simulink model "DG1"  (R2020a)
settings: Solver=VariableStepAuto  StartTime=0.0  StopTime=20  RelTol=1e-3
values from neighbouring files (symbols this model uses):
  cf1 = 50 * 1e-6    (= 5e-05)    [parameters.m]
  F1 = 0.75    [parameters.m]
  kic1 = 16e3    (= 16000)    [parameters.m]
  kiv1 = 390    [parameters.m]
  kpc1 = 10.5    [parameters.m]
  kpv1 = 0.05    [parameters.m]
  Lc1 = 0.35 * 1e-3    (= 0.00035)    [parameters.m]
  Lf1 = 1.35 * 1e-3    (= 0.00135)    [parameters.m]
  mp1 = 9.4 * 1e-5    (= 9.4e-05)    [parameters.m]
  nq1 = 1.3 * 1e-3    (= 0.0013)    [parameters.m]
  Rc1 = 0.03    [parameters.m]
  Rf1 = 0.1    [parameters.m]
  Tss = 2.5e-6    (= 2.5e-06)    [parameters.m]
  wb1 = 50 * 2 * pi    (= 314.159265359)    [parameters.m]
  wc1 = 31.41    [parameters.m]
  wcom = 0 * 2 * pi    (= 0)    [parameters.m]
undefined symbols (not defined in the file or in its folder): Lf
libraries: powerlib x12, powerlib_meascontrol x7
settings Model: Creator=derek  LastModifiedBy=derek

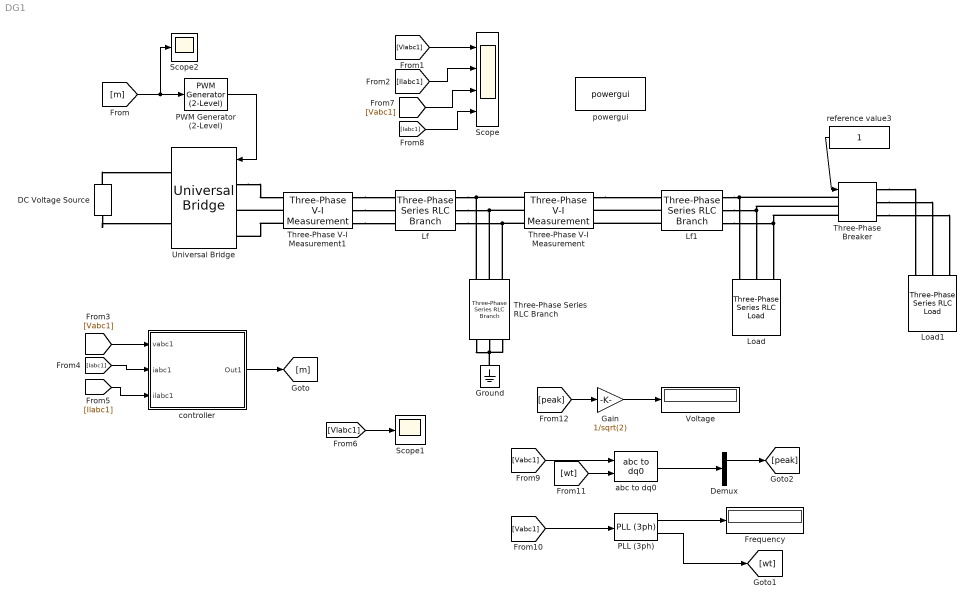
== system DG1 ==
  DC Voltage Source : powerlib/Electrical Sources/DC Voltage Source  Amplitude=600  Measurements=None
  Demux : Demux  Outputs=3
  Frequency : Display
  Gain : Gain  Gain=1/sqrt(2)
  Ground : powerlib/Elements/Ground  LConnTagsString=a
  Lf : powerlib/Elements/Three-Phase Series RLC Branch  LConnTagsString=A|B|C  RConnTagsString=A|B|C  BranchType=RL  Resistance=Rf1  Inductance=Lf1  Capacitance=Lf  Measurements=None
  Lf1 : powerlib/Elements/Three-Phase Series RLC Branch  LConnTagsString=A|B|C  RConnTagsString=A|B|C  BranchType=RL  Resistance=Rc1  Inductance=Lc1  Capacitance=Lf  Measurements=None
  Load : powerlib/Elements/Three-Phase Series RLC Load  LConnTagsString=A|B|C  Configuration=Y (grounded)  NominalVoltage=314  Vabc=[1e3 1e3 1e3]  Vabcp=[1e3 1e3 1e3]  NominalFrequency=50  UnbalancedPower=off  ActivePower=20e3  InductivePower=0  CapacitivePower=0  Pabc=[10e3 9e3 11e3]  QLabc=[100 90 110]  QCabc=[100 90 110]  Pabcp=[10e3 9e3 11e3]  QLabcp=[100 90 110]  QCabcp=[100 90 110]  Measurements=None  LoadType=constant Z
  Load1 : powerlib/Elements/Three-Phase Series RLC Load  LConnTagsString=A|B|C  Configuration=Y (grounded)  NominalVoltage=314  Vabc=[1e3 1e3 1e3]  Vabcp=[1e3 1e3 1e3]  NominalFrequency=50  UnbalancedPower=off  ActivePower=20e3  InductivePower=0  CapacitivePower=0  Pabc=[10e3 9e3 11e3]  QLabc=[100 90 110]  QCabc=[100 90 110]  Pabcp=[10e3 9e3 11e3]  QLabcp=[100 90 110]  QCabcp=[100 90 110]  Measurements=None  LoadType=constant Z
  PLL (3ph) : powerlib_meascontrol/PLL/PLL (3ph)  Fmin=45  Par_Init=[0, 50]  ParK=[180, 3200, 1]  TcD=1e-4  MaxRateChangeFreq=12  FilterCutOffFreq=25  Ts=Tss  AGC=on
  PWM Generator (2-Level) : powerlib_meascontrol/Pulse & Signal Generators/PWM Generator (2-Level)  ModulatorType=Three-phase bridge (6 pulses)  ModulatorMode=Unsynchronized  Fc=fsw  Pc=90  nF=27  MinMax="[ -1  1 ]"  SamplingTechnique=Natural  ModulatingSignals=off  m=0.8  Freq=60  Phase=0  Ts=Tss  ShowCarrierOutport=off
  Scope : Scope  NumInputPorts=4
  Scope1 : Scope
  Scope2 : Scope
  Three-Phase Series RLC Branch : powerlib/Elements/Three-Phase Series RLC Branch  LConnTagsString=A|B|C  RConnTagsString=A|B|C  BranchType=RC  Resistance=1e-6  Inductance=1e-3  Capacitance=cf1  Measurements=None
  Three-Phase V-I Measurement : powerlib/Measurements/Three-Phase V-I Measurement  VoltageMeasurement=phase-to-phase  SetLabelV=on  LabelV=Vabc1  Vpu=off  VpuLL=off  CurrentMeasurement=yes  SetLabelI=on  LabelI=Iabc1  Ipu=off  Pbase=100e6  Vbase=500e3  OutputType=Complex  PhasorSimulation=off  PSBequivalent=0
  Three-Phase V-I Measurement1 : powerlib/Measurements/Three-Phase V-I Measurement  VoltageMeasurement=phase-to-phase  SetLabelV=on  LabelV=Vlabc1  Vpu=off  VpuLL=off  CurrentMeasurement=yes  SetLabelI=on  LabelI=Ilabc1  Ipu=off  Pbase=100e6  Vbase=500e3  OutputType=Complex  PhasorSimulation=off  PSBequivalent=0
  Three-Phase Breaker : powerlib/Elements/Three-Phase Breaker  InitialState=open  SwitchA=on  SwitchB=on  SwitchC=on  SwitchTimes="[1/60  5/60]"  External=on  BreakerResistance=0.01  SnubberResistance=1e6  SnubberCapacitance=inf  Measurements=None
  Universal Bridge : powerlib/Power Electronics/Universal Bridge  Arms=3  SnubberResistance=1e5  SnubberCapacitance=inf  Device=IGBT / Diodes  Ron=1e-3  Lon=0  ForwardVoltages="[  0  0  ]"  ForwardVoltage=0  GTOparameters=[ 10e-6 , 20e-6 ]  IGBTparameters=[ 1e-6 , 2e-6 ]  Measurements=None  Measurements_2=None  converterType=Rectifier
  Voltage : Display
  abc to dq0 : powerlib_meascontrol/Transformations/abc to dq0  Alignment=90 degrees behind phase A axis
  controller : Subsystem
  powergui : powerlib/powergui  Priority=1  SimulationMode=Discrete  SampleTime=Tss  frequency=60  Iterations=50  frequencyindice=0  Pbase=100e6  ErrMax=1e-4  UnitsV=kV  UnitsW=MW  buscounter=0  FunctionMessages=off  echomessages=off  EnableUseOfTLC=off  CurrentSourceSwitches=off  DisableSnubberDevices=off  DisableRonSwitches=off  DisableVfSwitches=off  DisplayEquations=off  AutomaticDiscreteSolvers=off  SolverType=Tustin/Backward Euler (TBE)  Interpol=off  ExternalGateDelay=off  methode=off  Ts=100  x0status=blocks  SPID=on  SwTol=0  HookPort=off  NonlinearTolerance=0  nMaxIteration=15  ContinueOnMaxIteration=off  RestoreLinks=warning  ResistiveCurrentMeasurement=off  Frange=[0:2:500]  Ylog=off  Xlog=on  ShowGrid=off  save=off  variable=ZData  structure=0  ZoomFFT=off  StartTime=0.0  cycles=1  DisplayStyle=1  fundamental=60  FreqAxis=off  MaxFrequency=1000  frequencyindicesteady=1  RmsSteady=1  display=off
  reference value3 : Constant
  wires:
  [Ilabc1] -> Scope/2
  PWM Generator (2-Level)/1 -> Universal Bridge/1
  [m] -> Scope2/1, PWM Generator (2-Level)/1
  [Vlabc1] -> Scope/1
  [Vabc1] -> controller/1(vabc1)
  [Iabc1] -> controller/2(iabc1)
  [Ilabc1] -> controller/3(ilabc1)
  controller/1(Out1) -> [m]
  [Vlabc1] -> Scope1/1
  [Vabc1] -> Scope/3
  [Iabc1] -> Scope/4
  [Vabc1] -> PLL (3ph)/1
  Demux/1 -> [peak]
  [wt] -> abc to dq0/2
  PLL (3ph)/2 -> [wt]
  [Vabc1] -> abc to dq0/1
  Gain/1 -> Voltage/1
  abc to dq0/1 -> Demux/1
  [peak] -> Gain/1
  PLL (3ph)/1 -> Frequency/1
  reference value3/1 -> Three-Phase Breaker/1
  connections:
  Three-Phase Series RLC Branch/LConn3 -- Lf/RConn3 -- Three-Phase V-I Measurement/LConn3
  Three-Phase Series RLC Branch/LConn1 -- Lf/RConn1 -- Three-Phase V-I Measurement/LConn1
  Three-Phase Series RLC Branch/LConn2 -- Lf/RConn2 -- Three-Phase V-I Measurement/LConn2
  Three-Phase Series RLC Branch/RConn1 -- Ground/LConn1 -- Three-Phase Series RLC Branch/RConn3 -- Three-Phase Series RLC Branch/RConn2
  DC Voltage Source/RConn1 -- Universal Bridge/RConn1
  DC Voltage Source/LConn1 -- Universal Bridge/RConn2
  Three-Phase V-I Measurement1/RConn1 -- Lf/LConn1
  Three-Phase V-I Measurement1/RConn2 -- Lf/LConn2
  Three-Phase V-I Measurement1/RConn3 -- Lf/LConn3
  Universal Bridge/LConn1 -- Three-Phase V-I Measurement1/LConn1
  Three-Phase V-I Measurement1/LConn2 -- Universal Bridge/LConn2
  Three-Phase V-I Measurement1/LConn3 -- Universal Bridge/LConn3
  Three-Phase V-I Measurement/RConn1 -- Lf1/LConn1
  Lf1/LConn2 -- Three-Phase V-I Measurement/RConn2
  Lf1/LConn3 -- Three-Phase V-I Measurement/RConn3
  Lf1/RConn3 -- Three-Phase Breaker/LConn3 -- Load/LConn3
  Lf1/RConn2 -- Three-Phase Breaker/LConn2 -- Load/LConn2
  Lf1/RConn1 -- Three-Phase Breaker/LConn1 -- Load/LConn1
  Three-Phase Breaker/RConn2 -- Load1/LConn2
  Three-Phase Breaker/RConn3 -- Load1/LConn3
  Three-Phase Breaker/RConn1 -- Load1/LConn1

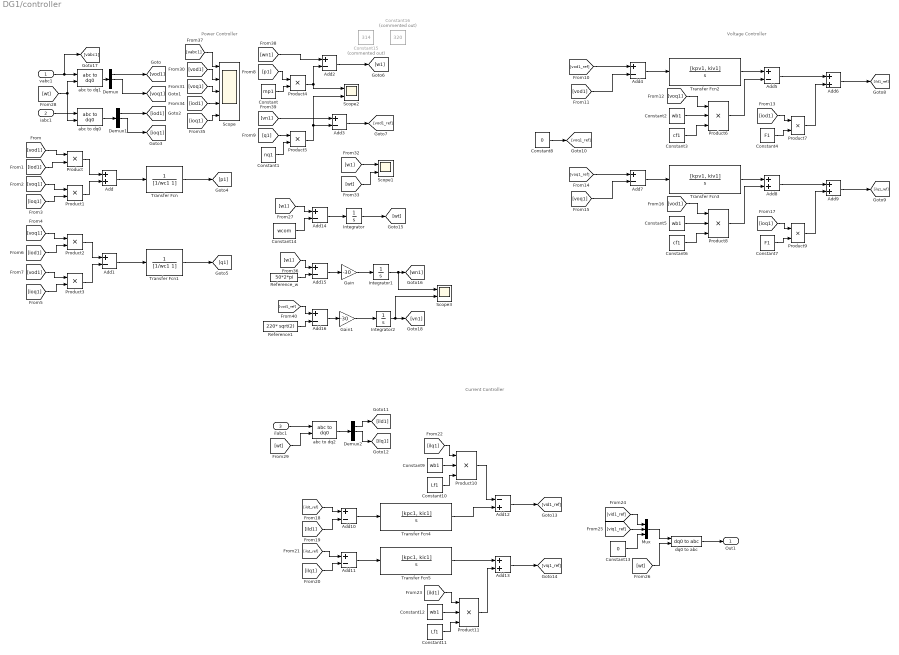
== system DG1/controller ==
  note: Voltage Controller
  note: Power Controller
  note: Current Controller
  vabc1 : Inport
  iabc1 : Inport  Port=2
  ilabc1 : Inport  Port=3
  Add{,6,8..9,13} (5 alike) : Sum
  Add{1..5,7,10..11,14..16} (11 alike) : Sum  Inputs=+-
  Add12 : Sum  Inputs=-+
  Constant : Constant  Value=mp1
  Constant1 : Constant  Value=nq1
  Constant10 : Constant  Value=Lf1
  Constant11 : Constant  Value=Lf1
  Constant{2,5,9,12} (4 alike) : Constant  Value=wb1
  Constant13 : Constant  Value=0
  Constant14 : Constant  Value=wcom  SampleTime=Tss
  Constant15 : Constant  Commented=on  Value=314
  Constant16 : Constant  Commented=on  Value=320
  Constant3 : Constant  Value=cf1
  Constant4 : Constant  Value=F1
  Constant6 : Constant  Value=cf1
  Constant7 : Constant  Value=F1
  Constant8 : Constant  Value=0
  Demux : Demux  Outputs=3
  Demux1 : Demux  Outputs=3
  Demux2 : Demux  Outputs=3
  Gain : Gain  Gain=-30
  Gain1 : Gain  Gain=-30
  Integrator : Integrator
  Integrator1 : Integrator  InitialCondition=50*2*pi
  Integrator2 : Integrator  InitialCondition=220*sqrt(2)
  Mux : Mux  Inputs=3
  Product{,1..5,7,9} (8 alike) : Product
  Product{6,8,10..11} (4 alike) : Product  Inputs=3
  Reference1 : Constant  Value=220* sqrt(2)  SampleTime=Tss
  Reference_w : Constant  Value=50*2*pi
  Scope : Scope  NumInputPorts=5
  Scope1 : Scope  NumInputPorts=2
  Scope2 : Scope  NumInputPorts=2
  Scope3 : Scope  NumInputPorts=2
  Transfer Fcn : TransferFcn  Denominator=[1/wc1 1]
  Transfer Fcn1 : TransferFcn  Denominator=[1/wc1 1]
  Transfer Fcn2 : TransferFcn  Numerator=[kpv1, kiv1]  Denominator=[1, 0]
  Transfer Fcn3 : TransferFcn  Numerator=[kpv1, kiv1]  Denominator=[1, 0]
  Transfer Fcn4 : TransferFcn  Numerator=[kpc1, kic1]  Denominator=[1, 0]
  Transfer Fcn5 : TransferFcn  Numerator=[kpc1, kic1]  Denominator=[1, 0]
  abc to dq0 : powerlib_meascontrol/Transformations/abc to dq0  Alignment=90 degrees behind phase A axis
  abc to dq1 : powerlib_meascontrol/Transformations/abc to dq0  Alignment=90 degrees behind phase A axis
  abc to dq2 : powerlib_meascontrol/Transformations/abc to dq0  Alignment=90 degrees behind phase A axis
  dq0 to abc : powerlib_meascontrol/Transformations/dq0 to abc  Alignment=90 degrees behind phase A axis
  Out1 : Outport
  wires:
  vabc1/1 -> [vabc1], abc to dq1/1
  iabc1/1 -> abc to dq0/1
  Demux/1 -> [vod1]
  Demux/2 -> [voq1]
  abc to dq1/1 -> Demux/1
  Demux1/2 -> [ioq1]
  Demux1/1 -> [iod1]
  abc to dq0/1 -> Demux1/1
  [vod1] -> Product/1
  [iod1] -> Product/2
  [voq1] -> Product1/1
  [ioq1] -> Product1/2
  Product/1 -> Add/1
  Product1/1 -> Add/2
  Add/1 -> Transfer Fcn/1
  Transfer Fcn/1 -> [p1]
  [voq1] -> Product2/1
  [iod1] -> Product2/2
  [vod1] -> Product3/1
  [ioq1] -> Product3/2
  Product2/1 -> Add1/1
  Product3/1 -> Add1/2
  Transfer Fcn1/1 -> [q1]
  Add1/1 -> Transfer Fcn1/1
  [p1] -> Product4/1
  Constant/1 -> Product4/2
  Product4/1 -> Scope2/1, Add2/2
  Add2/1 -> [w1]
  [q1] -> Product5/1
  Constant1/1 -> Product5/2
  Product5/1 -> Scope2/2, Add3/2
  Add3/1 -> [vod1_ref]
  [vod1_ref] -> Add4/1
  [vod1] -> Add4/2
  Add4/1 -> Transfer Fcn2/1
  Transfer Fcn2/1 -> Add5/1
  Constant2/1 -> Product6/2
  [voq1] -> Product6/1
  Constant3/1 -> Product6/3
  Product6/1 -> Add5/2
  Add5/1 -> Add6/1
  [iod1] -> Product7/1
  Constant4/1 -> Product7/2
  Product7/1 -> Add6/2
  Add6/1 -> [ild1_ref]
  Product8/1 -> Add8/2
  Constant6/1 -> Product8/3
  Add9/1 -> [ilq1_ref]
  Constant7/1 -> Product9/2
  Product9/1 -> Add9/2
  [ioq1] -> Product9/1
  Constant5/1 -> Product8/2
  [voq1] -> Add7/2
  [voq1_ref] -> Add7/1
  Add7/1 -> Transfer Fcn3/1
  Add8/1 -> Add9/1
  Transfer Fcn3/1 -> Add8/1
  [vod1] -> Product8/1
  Constant8/1 -> [voq1_ref]
  ilabc1/1 -> abc to dq2/1
  abc to dq2/1 -> Demux2/1
  Demux2/1 -> [ild1]
  Demux2/2 -> [ilq1]
  [ild1_ref] -> Add10/1
  [ild1] -> Add10/2
  [ilq1] -> Add11/2
  [ilq1_ref] -> Add11/1
  Add10/1 -> Transfer Fcn4/1
  Add11/1 -> Transfer Fcn5/1
  Transfer Fcn4/1 -> Add12/2
  [ilq1] -> Product10/1
  Constant9/1 -> Product10/2
  Constant10/1 -> Product10/3
  Product10/1 -> Add12/1
  Add12/1 -> [vid1_ref]
  Constant12/1 -> Product11/2
  [ild1] -> Product11/1
  Constant11/1 -> Product11/3
  Product11/1 -> Add13/2
  Transfer Fcn5/1 -> Add13/1
  Add13/1 -> [viq1_ref]
  [vid1_ref] -> Mux/1
  [viq1_ref] -> Mux/2
  Mux/1 -> dq0 to abc/1
  dq0 to abc/1 -> Out1/1
  [wt] -> dq0 to abc/2
  Constant13/1 -> Mux/3
  Constant14/1 -> Add14/2
  Add14/1 -> Integrator/1
  Integrator/1 -> [wt]
  [wt] -> abc to dq0/2, abc to dq1/2
  [wt] -> abc to dq2/2
  [w1] -> Scope1/1
  [wt] -> Scope1/2
  [ioq1] -> Scope/5
  [iod1] -> Scope/4
  [voq1] -> Scope/3
  [vod1] -> Scope/2
  [vabc1] -> Scope/1
  [w1] -> Add14/1
  [w1] -> Add15/1
  Reference_w/1 -> Add15/2
  Add15/1 -> Gain/1
  Integrator1/1 -> Scope3/1, [wn1]
  [vod1_ref] -> Add16/1
  Integrator2/1 -> Scope3/2, [vn1]
  Add16/1 -> Gain1/1
  Reference1/1 -> Add16/2
  Gain/1 -> Integrator1/1
  Gain1/1 -> Integrator2/1
  [vn1] -> Add3/1
  [wn1] -> Add2/1
